simulink model "Robot_daVinci_Simul_Kin"  (R2024b)
settings: Solver=VariableStepAuto  StartTime=0.0  StopTime=inf  RelTol=1e-3  EnableMultiTasking=on
libraries: Robot_daVinci_Lib x5
settings Model: Creator=jorgemartins  LastModifiedBy=raissare
settings SolverCC: AlgebraicLoopSolver=TrustRegion
settings DataIOCC: LimitDataPoints=on  ReturnWorkspaceOutputs=off
settings OptimizationCC: LifeSpan=inf
settings DebuggingCC: UnconnectedInputMsg=warning  UnconnectedOutputMsg=warning  UnconnectedLineMsg=warning  AllowSymbolicDim=off  SFUnexpectedBacktrackingDiag=warning  SFNoUnconditionalDefaultTransitionDiag=warning  SFExecutionAtInitializationDiag=none  ArithmeticOperatorsInVariantConditions=warning
settings ModelReferenceCC: EnableRefExpFcnMdlSchedulingChecks=on  PropagateSignalLabelsOutOfModel=off
settings SFSimCC: SimUseLocalCustomCode=off  CustomCodeUndefinedFunction=UseInterfaceOnly
settings RTWCC: RTWUseLocalCustomCode=off  GPUComputeCapability=3.5
settings CodeAppCC: StateflowObjectComments=on
settings GRTTargetCC: TargetLangStandard=C89/C90 (ANSI)
settings ConfigComp: CovMetricSettings=dw  CovSaveCumulativeToWorkspaceVar=on  CovSaveSingleToWorkspaceVar=on  CovExternalEMLEnable=off

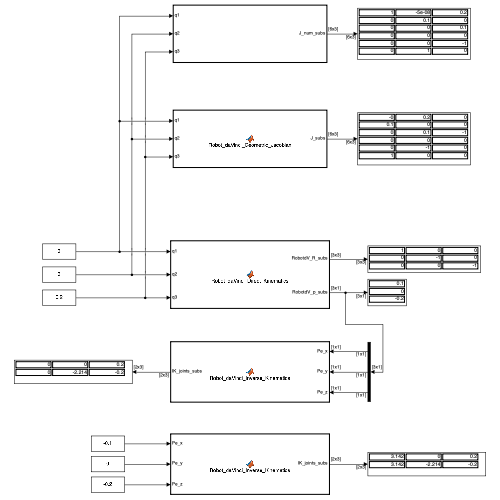
[thumbnail: Simulink's stored preview of the top-level diagram]
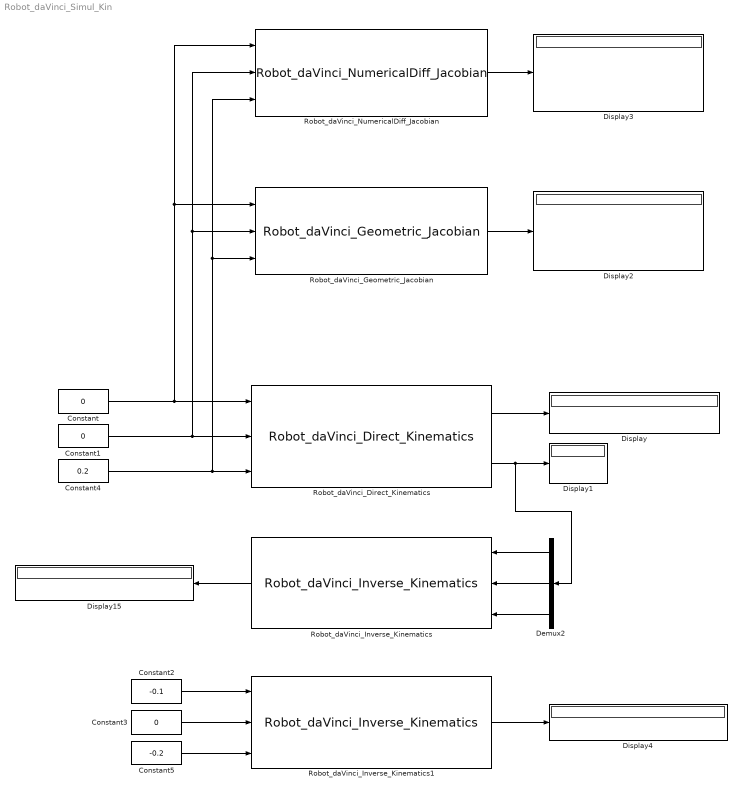
== system Robot_daVinci_Simul_Kin ==
  Constant : Constant  Value=0
  Constant1 : Constant  Value=0
  Constant2 : Constant  Value=-0.1
  Constant3 : Constant  Value=0
  Constant4 : Constant  Value=0.2
  Constant5 : Constant  Value=-0.2
  Demux2 : Demux  Outputs=3
  Display{,1..4,15} (6 alike) : Display
  Robot_daVinci_Direct_Kinematics : Robot_daVinci_Lib/Robot_daVinci_Direct_Kinematics  SystemSampleTime=-1  VariantActivationTime=update diagram  AllowFlexibleInterface=on  Latency=0  AutoFrameSizeCalculation=off
  Robot_daVinci_Geometric_Jacobian : Robot_daVinci_Lib/Robot_daVinci_Geometric_Jacobian  SystemSampleTime=-1  VariantActivationTime=update diagram  AllowFlexibleInterface=on  Latency=0  AutoFrameSizeCalculation=off
  Robot_daVinci_Inverse_Kinematics : Robot_daVinci_Lib/Robot_daVinci_Inverse_Kinematics  SystemSampleTime=-1  VariantActivationTime=update diagram  AllowFlexibleInterface=on  Latency=0  AutoFrameSizeCalculation=off
  Robot_daVinci_Inverse_Kinematics1 : Robot_daVinci_Lib/Robot_daVinci_Inverse_Kinematics  SystemSampleTime=-1  VariantActivationTime=update diagram  AllowFlexibleInterface=on  Latency=0  AutoFrameSizeCalculation=off
  Robot_daVinci_NumericalDiff_Jacobian : Robot_daVinci_Lib/Robot_daVinci_NumericalDiff_Jacobian  SystemSampleTime=-1  VariantActivationTime=update diagram  AllowFlexibleInterface=on  Latency=0  AutoFrameSizeCalculation=off
  wires:
  Robot_daVinci_Direct_Kinematics/1 -> Display/1
  Constant/1 -> Robot_daVinci_Direct_Kinematics/1, Robot_daVinci_NumericalDiff_Jacobian/1, Robot_daVinci_Geometric_Jacobian/1
  Constant4/1 -> Robot_daVinci_NumericalDiff_Jacobian/3, Robot_daVinci_Geometric_Jacobian/3, Robot_daVinci_Direct_Kinematics/3
  Constant1/1 -> Robot_daVinci_NumericalDiff_Jacobian/2, Robot_daVinci_Geometric_Jacobian/2, Robot_daVinci_Direct_Kinematics/2
  Robot_daVinci_Geometric_Jacobian/1 -> Display2/1
  Robot_daVinci_NumericalDiff_Jacobian/1 -> Display3/1
  Robot_daVinci_Direct_Kinematics/2 -> Display1/1, Demux2/1
  Demux2/2 -> Robot_daVinci_Inverse_Kinematics/2
  Demux2/1 -> Robot_daVinci_Inverse_Kinematics/1
  Demux2/3 -> Robot_daVinci_Inverse_Kinematics/3
  Robot_daVinci_Inverse_Kinematics/1 -> Display15/1
  Robot_daVinci_Inverse_Kinematics1/1 -> Display4/1
  Constant3/1 -> Robot_daVinci_Inverse_Kinematics1/2
  Constant2/1 -> Robot_daVinci_Inverse_Kinematics1/1
  Constant5/1 -> Robot_daVinci_Inverse_Kinematics1/3
